simulink subsystem "Ground"  (R2026a)
settings: Solver=VariableStepAuto
undefined symbols (not defined in the file): r_leg_1, r_leg_2, r_leg_3, r_leg_4
libraries: matrix_library x8, simulink x2
settings Model: Creator=ripro  LastModifiedBy=ripro

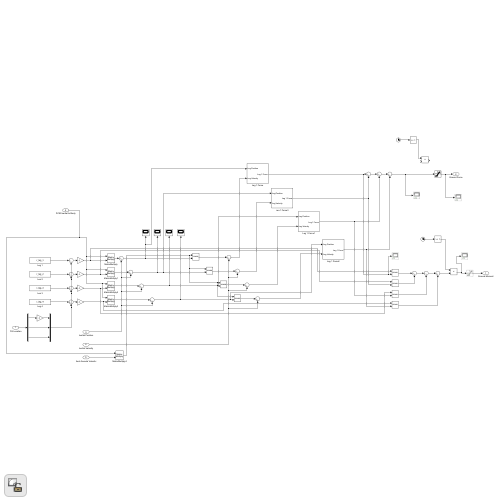
[thumbnail: Simulink's stored preview of the top-level diagram]
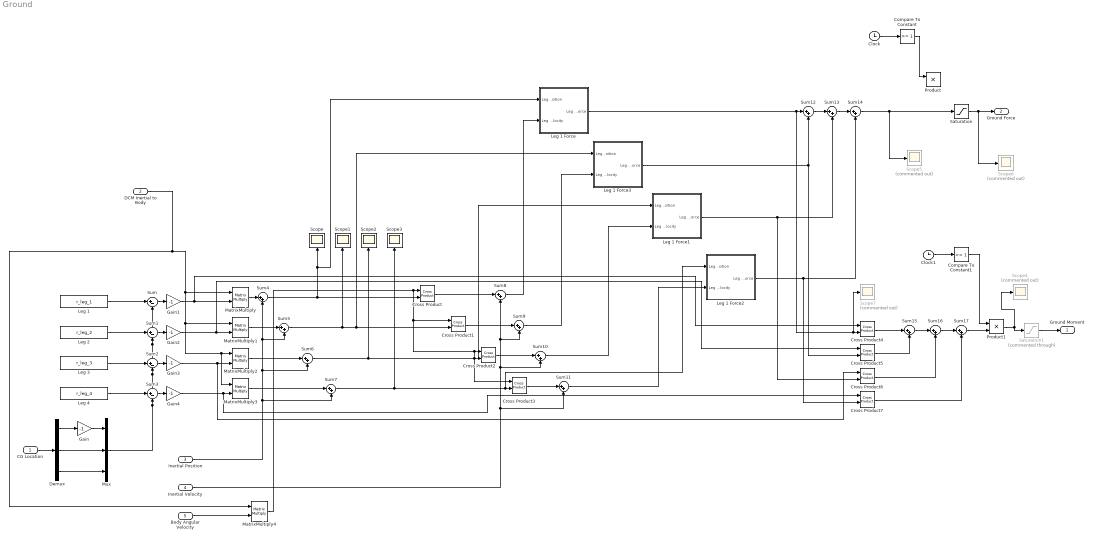
== system Ground ==
  CG Location : Inport
  DCM Inertial to Body : Inport  Port=2
  Inertial Position : Inport  Port=3
  Inertial Velocity : Inport  Port=4
  Body Angular Velocity : Inport  Port=5
  Clock : Clock
  Clock1 : Clock
  Compare To Constant : simulink/Logic and Bit Operations/Compare To Constant  relop=>=  const=1  OutDataTypeStr=boolean
  Compare To Constant1 : simulink/Logic and Bit Operations/Compare To Constant  relop=>=  const=1  OutDataTypeStr=boolean
  Cross Product{,1..7} (8 alike) : matrix_library/Cross Product
  Demux : Demux  Outputs=3
  Gain{,1..4} (5 alike) : Gain  Gain=-1
  Leg 1 : Constant  Value=r_leg_1
  Leg 1 Force : Subsystem
  Leg 1 Force1 : Subsystem
  Leg 1 Force2 : Subsystem
  Leg 1 Force3 : Subsystem
  Leg 2 : Constant  Value=r_leg_2
  Leg 3 : Constant  Value=r_leg_3
  Leg 4 : Constant  Value=r_leg_4
  MatrixMultiply{,1..4} (5 alike) : Product  Multiplication=Matrix(*)
  Mux : Mux  Inputs=3
  Product : Product
  Product1 : Product
  Saturation : Saturate  UpperLimit=inf  LowerLimit=0
  Saturation1 : Saturate  Commented=through  UpperLimit=inf  LowerLimit=0
  Scope{,1..3} (4 alike) : Scope
      Scope settings: ActiveDisplayYMinimum=-19.811154048207108  ActiveDisplayYMaximum=167.31101950999761  DataLoggingVariableName=ScopeData24
      Scope1 settings: ActiveDisplayYMinimum=182.10765195211306  ActiveDisplayYMaximum=183.93696889205802  DataLoggingVariableName=ScopeData30
      Scope2 settings: DataLoggingVariableName=ScopeData31
      Scope3 settings: DataLoggingVariableName=ScopeData42
  Scope{4..7} (4 alike) : Scope  Commented=on
      Scope4 settings: ActiveDisplayYMinimum=-3.0293963365637429E+7  ActiveDisplayYMaximum=2.2731893212350109E+8  DataLoggingVariableName=ScopeData43
      Scope5 settings: ActiveDisplayYMinimum=-31343.151613259419  ActiveDisplayYMaximum=282088.36451933486  DataLoggingVariableName=ScopeData44
      Scope6 settings: ActiveDisplayYMinimum=-136.62925150266653  ActiveDisplayYMaximum=1229.6632635239991  DataLoggingVariableName=ScopeData45
      Scope7 settings: ActiveDisplayYMinimum=-3.5823523450793636E+8  ActiveDisplayYMaximum=5.8466661508525646E+8  DataLoggingVariableName=ScopeData61
  Sum{,1..3} (4 alike) : Sum  Inputs=|+-
  Sum{4..17} (14 alike) : Sum  Inputs=|++
  Ground Moment : Outport
  Ground Force : Outport  Port=2
  wires:
  Demux/2 -> Mux/2
  Demux/3 -> Mux/3
  Leg 1/1 -> Sum/1
  Leg 2/1 -> Sum1/1
  Leg 3/1 -> Sum2/1
  Leg 4/1 -> Sum3/1
  Mux/1 -> Sum2/2, Sum/2, Sum1/2, Sum3/2
  Sum/1 -> Gain1/1
  DCM Inertial to Body/1 -> MatrixMultiply/1, MatrixMultiply2/1, MatrixMultiply3/1, MatrixMultiply1/1, MatrixMultiply4/1
  Sum1/1 -> Gain2/1
  Sum2/1 -> Gain3/1
  Sum3/1 -> Gain4/1
  MatrixMultiply3/1 -> Sum7/1
  MatrixMultiply2/1 -> Sum6/1
  MatrixMultiply1/1 -> Sum5/1
  MatrixMultiply/1 -> Sum4/1
  Inertial Position/1 -> Sum4/2, Sum5/2, Sum6/2, Sum7/2
  Sum4/1 -> Cross Product/2, Leg 1 Force/1(Leg Position), Scope/1
  Sum5/1 -> Scope1/1, Cross Product1/2, Leg 1 Force3/1(Leg Position)
  Sum6/1 -> Scope2/1, Cross Product2/2, Leg 1 Force1/1(Leg Position)
  Sum7/1 -> Scope3/1, Cross Product3/2, Leg 1 Force2/1(Leg Position)
  Body Angular Velocity/1 -> MatrixMultiply4/2
  MatrixMultiply4/1 -> Cross Product/1, Cross Product2/1, Cross Product3/1, Cross Product1/1
  Cross Product/1 -> Sum8/1
  Cross Product1/1 -> Sum9/1
  Cross Product2/1 -> Sum10/1
  Cross Product3/1 -> Sum11/1
  Inertial Velocity/1 -> Sum8/2, Sum9/2, Sum10/2, Sum11/2
  Leg 1 Force/1(Leg 1 Force) -> Sum12/1, Cross Product4/2, Scope7/1
  Leg 1 Force3/1(Leg 1 Force) -> Sum12/2, Cross Product5/2
  Sum12/1 -> Sum13/1
  Leg 1 Force1/1(Leg 1 Force) -> Sum13/2, Cross Product6/2
  Sum13/1 -> Sum14/1
  Leg 1 Force2/1(Leg 1 Force) -> Sum14/2, Cross Product7/2
  Cross Product4/1 -> Sum15/1
  Sum15/1 -> Sum16/1
  Cross Product5/1 -> Sum15/2
  Cross Product6/1 -> Sum16/2
  Sum16/1 -> Sum17/1
  Cross Product7/1 -> Sum17/2
  Sum8/1 -> Leg 1 Force/2(Leg Velocity)
  Sum9/1 -> Leg 1 Force3/2(Leg Velocity)
  Sum10/1 -> Leg 1 Force1/2(Leg Velocity)
  Sum11/1 -> Leg 1 Force2/2(Leg Velocity)
  Saturation/1 -> Scope6/1, Ground Force/1
  Saturation1/1 -> Ground Moment/1
  Gain/1 -> Mux/1
  Gain1/1 -> MatrixMultiply/2, Cross Product4/1
  Gain2/1 -> MatrixMultiply1/2, Cross Product5/1
  Gain3/1 -> MatrixMultiply2/2, Cross Product6/1
  Gain4/1 -> MatrixMultiply3/2, Cross Product7/1
  Sum14/1 -> Scope5/1, Saturation/1
  Clock1/1 -> Compare To Constant1/1
  Compare To Constant1/1 -> Product1/1
  Sum17/1 -> Product1/2
  Product1/1 -> Saturation1/1, Scope4/1
  CG Location/1 -> Demux/1
  Demux/1 -> Gain/1
  Clock/1 -> Compare To Constant/1
  Compare To Constant/1 -> Product/1

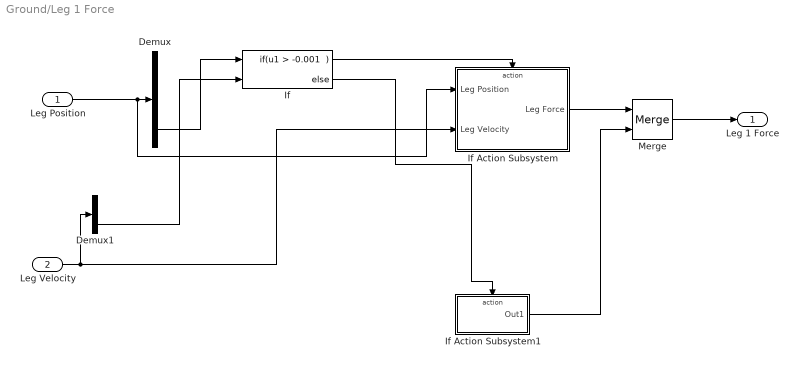
== system Ground/Leg 1 Force ==
  Leg Position : Inport
  Leg Velocity : Inport  Port=2
  Demux : Demux  Outputs=3
  Demux1 : Demux  Outputs=3
  If : If  NumInputs=2  IfExpression=u1 > -0.001
  If Action Subsystem : Subsystem  TreatAsAtomicUnit=on
  If Action Subsystem1 : Subsystem  TreatAsAtomicUnit=on
  Merge : Merge
  Leg 1 Force : Outport
  wires:
  Demux1/3 -> If/2
  Demux/3 -> If/1
  If/1 -> If Action Subsystem/Action
  Leg Velocity/1 -> If Action Subsystem/2(Leg Velocity), Demux1/1
  Merge/1 -> Leg 1 Force/1
  If Action Subsystem1/1(Out1) -> Merge/2
  If Action Subsystem/1(Leg Force) -> Merge/1
  If/2 -> If Action Subsystem1/Action
  Leg Position/1 -> Demux/1, If Action Subsystem/1(Leg Position)

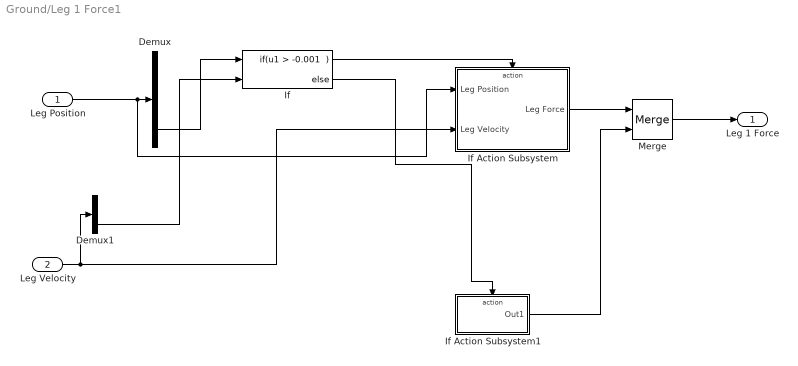
== system Ground/Leg 1 Force1 ==
  Leg Position : Inport
  Leg Velocity : Inport  Port=2
  Demux : Demux  Outputs=3
  Demux1 : Demux  Outputs=3
  If : If  NumInputs=2  IfExpression=u1 > -0.001
  If Action Subsystem : Subsystem  TreatAsAtomicUnit=on
  If Action Subsystem1 : Subsystem  TreatAsAtomicUnit=on
  Merge : Merge
  Leg 1 Force : Outport
  wires:
  Demux1/3 -> If/2
  Demux/3 -> If/1
  If/1 -> If Action Subsystem/Action
  Leg Velocity/1 -> If Action Subsystem/2(Leg Velocity), Demux1/1
  Merge/1 -> Leg 1 Force/1
  If Action Subsystem1/1(Out1) -> Merge/2
  If Action Subsystem/1(Leg Force) -> Merge/1
  If/2 -> If Action Subsystem1/Action
  Leg Position/1 -> Demux/1, If Action Subsystem/1(Leg Position)

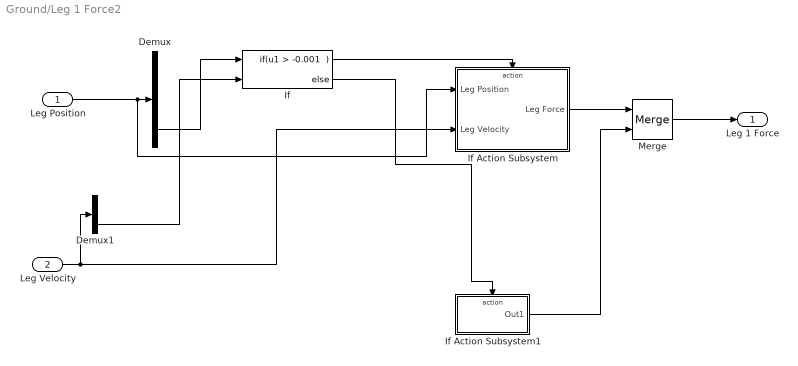
== system Ground/Leg 1 Force2 ==
  Leg Position : Inport
  Leg Velocity : Inport  Port=2
  Demux : Demux  Outputs=3
  Demux1 : Demux  Outputs=3
  If : If  NumInputs=2  IfExpression=u1 > -0.001
  If Action Subsystem : Subsystem  TreatAsAtomicUnit=on
  If Action Subsystem1 : Subsystem  TreatAsAtomicUnit=on
  Merge : Merge
  Leg 1 Force : Outport
  wires:
  Demux1/3 -> If/2
  Demux/3 -> If/1
  If/1 -> If Action Subsystem/Action
  Leg Velocity/1 -> If Action Subsystem/2(Leg Velocity), Demux1/1
  Merge/1 -> Leg 1 Force/1
  If Action Subsystem1/1(Out1) -> Merge/2
  If Action Subsystem/1(Leg Force) -> Merge/1
  If/2 -> If Action Subsystem1/Action
  Leg Position/1 -> Demux/1, If Action Subsystem/1(Leg Position)

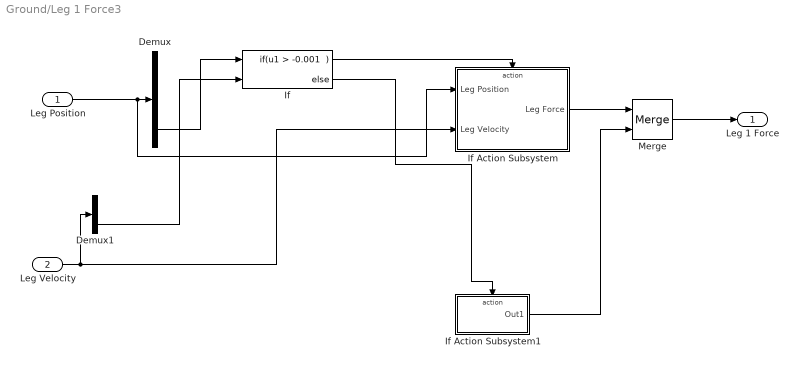
== system Ground/Leg 1 Force3 ==
  Leg Position : Inport
  Leg Velocity : Inport  Port=2
  Demux : Demux  Outputs=3
  Demux1 : Demux  Outputs=3
  If : If  NumInputs=2  IfExpression=u1 > -0.001
  If Action Subsystem : Subsystem  TreatAsAtomicUnit=on
  If Action Subsystem1 : Subsystem  TreatAsAtomicUnit=on
  Merge : Merge
  Leg 1 Force : Outport
  wires:
  Demux1/3 -> If/2
  Demux/3 -> If/1
  If/1 -> If Action Subsystem/Action
  Leg Velocity/1 -> If Action Subsystem/2(Leg Velocity), Demux1/1
  Merge/1 -> Leg 1 Force/1
  If Action Subsystem1/1(Out1) -> Merge/2
  If Action Subsystem/1(Leg Force) -> Merge/1
  If/2 -> If Action Subsystem1/Action
  Leg Position/1 -> Demux/1, If Action Subsystem/1(Leg Position)

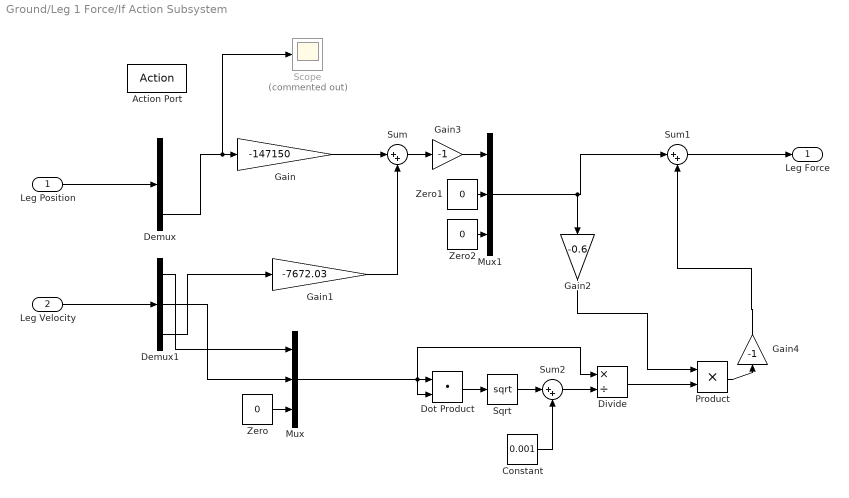
== system Ground/Leg 1 Force/If Action Subsystem ==
  Leg Position : Inport
  Leg Velocity : Inport  Port=2
  Action Port : ActionPort
  Constant : Constant  Value=0.001
  Demux : Demux  Outputs=3
  Demux1 : Demux  Outputs=3
  Divide : Product  Inputs=*/
  Dot Product : DotProduct  OutDataTypeStr=Inherit: Inherit via internal rule
  Gain : Gain  Gain=-147150
  Gain1 : Gain  Gain=-7672.03
  Gain2 : Gain  Gain=-0.6
  Gain3 : Gain  Gain=-1
  Gain4 : Gain  Gain=-1
  Mux : Mux  Inputs=3
  Mux1 : Mux  Inputs=3
  Product : Product
  Scope : Scope  Commented=on
      settings: ActiveDisplayYMinimum=-1  ActiveDisplayYMaximum=1  DataLoggingVariableName=ScopeData69
  Sqrt : Sqrt
  Sum : Sum  Inputs=|++
  Sum1 : Sum  Inputs=|++
  Sum2 : Sum  Inputs=|++
  Zero : Constant  Value=0  OutDataTypeStr=Inherit: Inherit via back propagation
  Zero1 : Constant  Value=0  OutDataTypeStr=Inherit: Inherit via back propagation
  Zero2 : Constant  Value=0  OutDataTypeStr=Inherit: Inherit via back propagation
  Leg Force : Outport
  wires:
  Gain4/1 -> Sum1/2
  Gain3/1 -> Mux1/1
  Zero/1 -> Mux/3
  Demux/3 -> Gain/1, Scope/1
  Mux1/1 -> Gain2/1, Sum1/1
  Zero2/1 -> Mux1/3
  Zero1/1 -> Mux1/2
  Sum/1 -> Gain3/1
  Constant/1 -> Sum2/2
  Sum2/1 -> Divide/2
  Sqrt/1 -> Sum2/1
  Sum1/1 -> Leg Force/1
  Product/1 -> Gain4/1
  Gain2/1 -> Product/1
  Divide/1 -> Product/2
  Dot Product/1 -> Sqrt/1
  Mux/1 -> Divide/1, Dot Product/1, Dot Product/2
  Demux1/1 -> Mux/1
  Demux1/2 -> Mux/2
  Demux1/3 -> Gain1/1
  Gain1/1 -> Sum/2
  Gain/1 -> Sum/1
  Leg Velocity/1 -> Demux1/1
  Leg Position/1 -> Demux/1

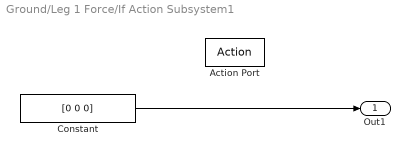
== system Ground/Leg 1 Force/If Action Subsystem1 ==
  Action Port : ActionPort
  Constant : Constant  Value=[0 0 0]
  Out1 : Outport
  wires:
  Constant/1 -> Out1/1

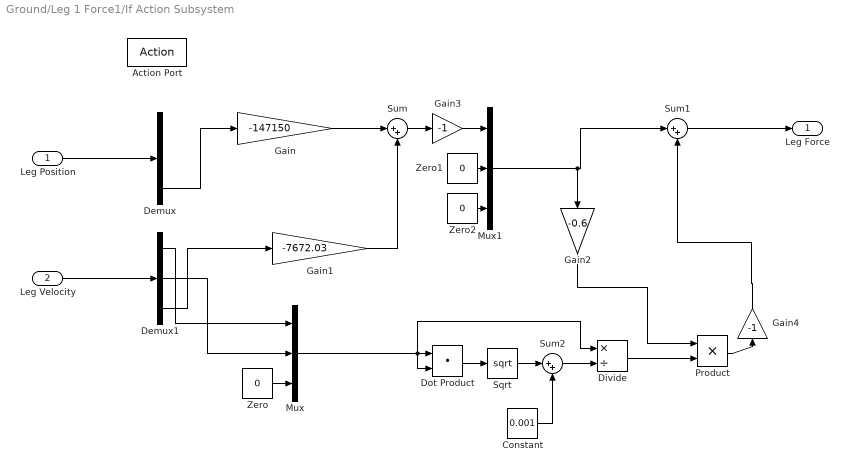
== system Ground/Leg 1 Force1/If Action Subsystem ==
  Leg Position : Inport
  Leg Velocity : Inport  Port=2
  Action Port : ActionPort
  Constant : Constant  Value=0.001
  Demux : Demux  Outputs=3
  Demux1 : Demux  Outputs=3
  Divide : Product  Inputs=*/
  Dot Product : DotProduct  OutDataTypeStr=Inherit: Inherit via internal rule
  Gain : Gain  Gain=-147150
  Gain1 : Gain  Gain=-7672.03
  Gain2 : Gain  Gain=-0.6
  Gain3 : Gain  Gain=-1
  Gain4 : Gain  Gain=-1
  Mux : Mux  Inputs=3
  Mux1 : Mux  Inputs=3
  Product : Product
  Sqrt : Sqrt
  Sum : Sum  Inputs=|++
  Sum1 : Sum  Inputs=|++
  Sum2 : Sum  Inputs=|++
  Zero : Constant  Value=0  OutDataTypeStr=Inherit: Inherit via back propagation
  Zero1 : Constant  Value=0  OutDataTypeStr=Inherit: Inherit via back propagation
  Zero2 : Constant  Value=0  OutDataTypeStr=Inherit: Inherit via back propagation
  Leg Force : Outport
  wires:
  Gain4/1 -> Sum1/2
  Gain3/1 -> Mux1/1
  Zero/1 -> Mux/3
  Demux/3 -> Gain/1
  Mux1/1 -> Gain2/1, Sum1/1
  Zero2/1 -> Mux1/3
  Zero1/1 -> Mux1/2
  Sum/1 -> Gain3/1
  Constant/1 -> Sum2/2
  Sum2/1 -> Divide/2
  Sqrt/1 -> Sum2/1
  Sum1/1 -> Leg Force/1
  Product/1 -> Gain4/1
  Gain2/1 -> Product/1
  Divide/1 -> Product/2
  Dot Product/1 -> Sqrt/1
  Mux/1 -> Divide/1, Dot Product/1, Dot Product/2
  Demux1/1 -> Mux/1
  Demux1/2 -> Mux/2
  Demux1/3 -> Gain1/1
  Gain1/1 -> Sum/2
  Gain/1 -> Sum/1
  Leg Velocity/1 -> Demux1/1
  Leg Position/1 -> Demux/1

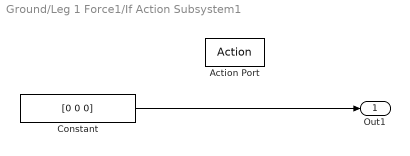
== system Ground/Leg 1 Force1/If Action Subsystem1 ==
  Action Port : ActionPort
  Constant : Constant  Value=[0 0 0]
  Out1 : Outport
  wires:
  Constant/1 -> Out1/1

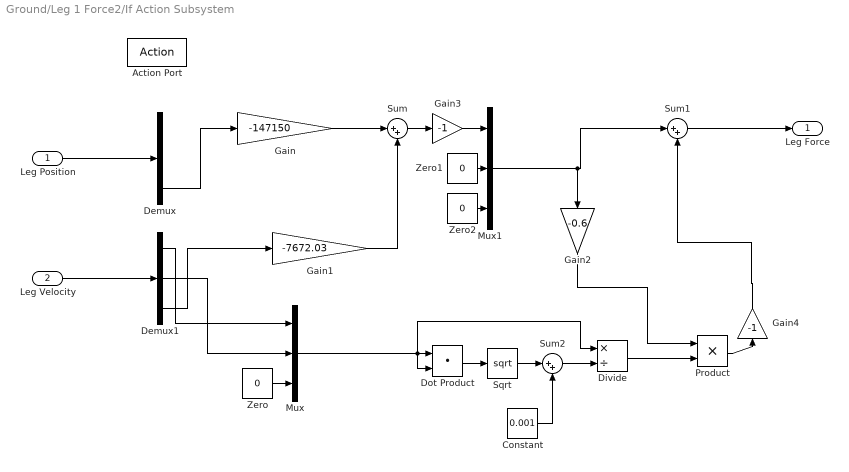
== system Ground/Leg 1 Force2/If Action Subsystem ==
  Leg Position : Inport
  Leg Velocity : Inport  Port=2
  Action Port : ActionPort
  Constant : Constant  Value=0.001
  Demux : Demux  Outputs=3
  Demux1 : Demux  Outputs=3
  Divide : Product  Inputs=*/
  Dot Product : DotProduct  OutDataTypeStr=Inherit: Inherit via internal rule
  Gain : Gain  Gain=-147150
  Gain1 : Gain  Gain=-7672.03
  Gain2 : Gain  Gain=-0.6
  Gain3 : Gain  Gain=-1
  Gain4 : Gain  Gain=-1
  Mux : Mux  Inputs=3
  Mux1 : Mux  Inputs=3
  Product : Product
  Sqrt : Sqrt
  Sum : Sum  Inputs=|++
  Sum1 : Sum  Inputs=|++
  Sum2 : Sum  Inputs=|++
  Zero : Constant  Value=0  OutDataTypeStr=Inherit: Inherit via back propagation
  Zero1 : Constant  Value=0  OutDataTypeStr=Inherit: Inherit via back propagation
  Zero2 : Constant  Value=0  OutDataTypeStr=Inherit: Inherit via back propagation
  Leg Force : Outport
  wires:
  Gain4/1 -> Sum1/2
  Gain3/1 -> Mux1/1
  Zero/1 -> Mux/3
  Demux/3 -> Gain/1
  Mux1/1 -> Gain2/1, Sum1/1
  Zero2/1 -> Mux1/3
  Zero1/1 -> Mux1/2
  Sum/1 -> Gain3/1
  Constant/1 -> Sum2/2
  Sum2/1 -> Divide/2
  Sqrt/1 -> Sum2/1
  Sum1/1 -> Leg Force/1
  Product/1 -> Gain4/1
  Gain2/1 -> Product/1
  Divide/1 -> Product/2
  Dot Product/1 -> Sqrt/1
  Mux/1 -> Divide/1, Dot Product/1, Dot Product/2
  Demux1/1 -> Mux/1
  Demux1/2 -> Mux/2
  Demux1/3 -> Gain1/1
  Gain1/1 -> Sum/2
  Gain/1 -> Sum/1
  Leg Velocity/1 -> Demux1/1
  Leg Position/1 -> Demux/1

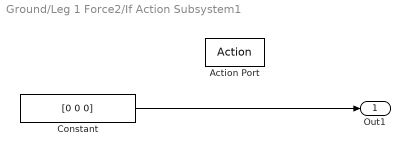
== system Ground/Leg 1 Force2/If Action Subsystem1 ==
  Action Port : ActionPort
  Constant : Constant  Value=[0 0 0]
  Out1 : Outport
  wires:
  Constant/1 -> Out1/1

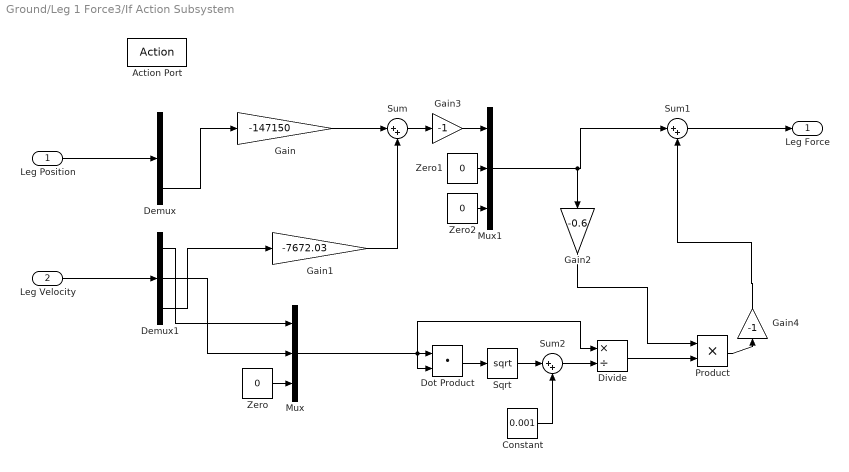
== system Ground/Leg 1 Force3/If Action Subsystem ==
  Leg Position : Inport
  Leg Velocity : Inport  Port=2
  Action Port : ActionPort
  Constant : Constant  Value=0.001
  Demux : Demux  Outputs=3
  Demux1 : Demux  Outputs=3
  Divide : Product  Inputs=*/
  Dot Product : DotProduct  OutDataTypeStr=Inherit: Inherit via internal rule
  Gain : Gain  Gain=-147150
  Gain1 : Gain  Gain=-7672.03
  Gain2 : Gain  Gain=-0.6
  Gain3 : Gain  Gain=-1
  Gain4 : Gain  Gain=-1
  Mux : Mux  Inputs=3
  Mux1 : Mux  Inputs=3
  Product : Product
  Sqrt : Sqrt
  Sum : Sum  Inputs=|++
  Sum1 : Sum  Inputs=|++
  Sum2 : Sum  Inputs=|++
  Zero : Constant  Value=0  OutDataTypeStr=Inherit: Inherit via back propagation
  Zero1 : Constant  Value=0  OutDataTypeStr=Inherit: Inherit via back propagation
  Zero2 : Constant  Value=0  OutDataTypeStr=Inherit: Inherit via back propagation
  Leg Force : Outport
  wires:
  Gain4/1 -> Sum1/2
  Gain3/1 -> Mux1/1
  Zero/1 -> Mux/3
  Demux/3 -> Gain/1
  Mux1/1 -> Gain2/1, Sum1/1
  Zero2/1 -> Mux1/3
  Zero1/1 -> Mux1/2
  Sum/1 -> Gain3/1
  Constant/1 -> Sum2/2
  Sum2/1 -> Divide/2
  Sqrt/1 -> Sum2/1
  Sum1/1 -> Leg Force/1
  Product/1 -> Gain4/1
  Gain2/1 -> Product/1
  Divide/1 -> Product/2
  Dot Product/1 -> Sqrt/1
  Mux/1 -> Divide/1, Dot Product/1, Dot Product/2
  Demux1/1 -> Mux/1
  Demux1/2 -> Mux/2
  Demux1/3 -> Gain1/1
  Gain1/1 -> Sum/2
  Gain/1 -> Sum/1
  Leg Velocity/1 -> Demux1/1
  Leg Position/1 -> Demux/1

== system Ground/Leg 1 Force3/If Action Subsystem1 ==
  Action Port : ActionPort
  Constant : Constant  Value=[0 0 0]
  Out1 : Outport
  wires:
  Constant/1 -> Out1/1
